simulink subsystem "multi_vehicle_test_subsystem"  (R2025a)
settings: Solver=VariableStepAuto  StartTime=0.0  StopTime=10.0  RelTol=1e-3
libraries: dspstat3 x1
settings Model: Creator=sanborkl  LastModifiedBy=admin

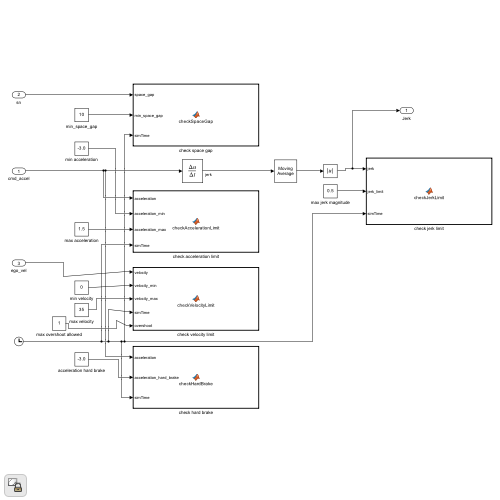
[thumbnail: Simulink's stored preview of the top-level diagram]
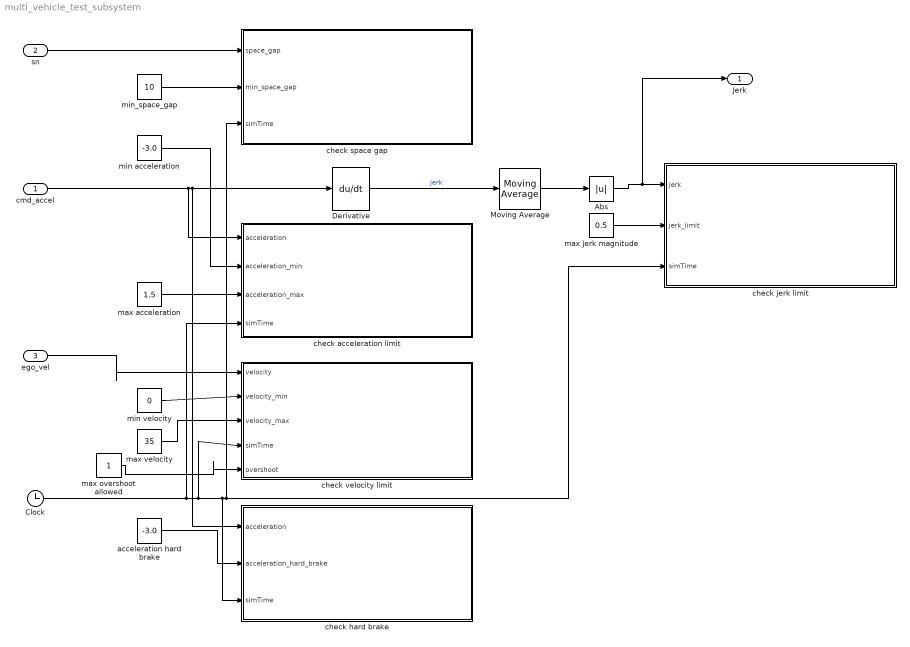
== system multi_vehicle_test_subsystem ==
  cmd_accel : Inport
  sn : Inport  Port=2
  ego_vel : Inport  Port=3
  Abs : Abs  ZeroCross=off  SaturateOnIntegerOverflow=off
  Clock : Clock
  Derivative : Derivative
  Moving Average : dspstat3/Moving Average  Method=Sliding window  ForgettingFactorPort=off  SpecifyWindowLength=on  WindowLength=10  OverlapLength=9  AllowArbitraryInputLength=off  ForgettingFactor=0.9  SimulateUsing=Interpreted execution
  acceleration hard brake : Constant  Value=-3.0
  check acceleration limit : MATLAB Function  TreatAsAtomicUnit=on
  check hard brake : MATLAB Function  TreatAsAtomicUnit=on
  check jerk limit : MATLAB Function  TreatAsAtomicUnit=on
  check space gap : MATLAB Function  TreatAsAtomicUnit=on
  check velocity limit : MATLAB Function  TreatAsAtomicUnit=on
  max acceleration : Constant  Value=1.5
  max jerk magnitude : Constant  Value=0.5
  max overshoot allowed : Constant
  max velocity : Constant  Value=35
  min acceleration : Constant  Value=-3.0
  min velocity : Constant  Value=0
  min_space_gap : Constant  Value=10
  Jerk : Outport
  wires:
  Moving Average/1 -> Abs/1
  min acceleration/1 -> check acceleration limit/2(acceleration_min)
  min_space_gap/1 -> check space gap/2(min_space_gap)
  Clock/1 -> check space gap/3(simTime), check jerk limit/3(simTime), check hard brake/3(simTime), check velocity limit/4(simTime), check acceleration limit/4(simTime)
  sn/1 -> check space gap/1(space_gap)
  ego_vel/1 -> check velocity limit/1(velocity)
  cmd_accel/1 -> Derivative/1, check hard brake/1(acceleration), check acceleration limit/1(acceleration)
  Derivative/1 -> Moving Average/1  "jerk"
  Abs/1 -> Jerk/1, check jerk limit/1(jerk)
  acceleration hard brake/1 -> check hard brake/2(acceleration_hard_brake)
  max acceleration/1 -> check acceleration limit/3(acceleration_max)
  max velocity/1 -> check velocity limit/3(velocity_max)
  min velocity/1 -> check velocity limit/2(velocity_min)
  max jerk magnitude/1 -> check jerk limit/2(jerk_limit)
  max overshoot allowed/1 -> check velocity limit/5(overshoot)

== matlab function multi_vehicle_test_subsystem/check jerk limit ==
  data: jerk input; jerk_limit input; simTime input
function checkJerkLimit(jerk, jerk_limit, simTime)
%#codegen
coder.extrinsic('disp', 'sprintf');

if abs(jerk) > jerk_limit
    msg = sprintf('Warning: Jerk exceeded limit: %.3f > %.3f at t=%.3f', ...
                  abs(jerk), jerk_limit, simTime);
    disp(msg);
end
end

== matlab function multi_vehicle_test_subsystem/check acceleration limit ==
  data: acceleration input; acceleration_min input; acceleration_max input; simTime input
function checkAccelerationLimit(acceleration, acceleration_min, acceleration_max, simTime)
%#codegen
coder.extrinsic('disp', 'sprintf');

if acceleration < acceleration_min || acceleration > acceleration_max
    msg = sprintf('Warning: Acceleration outside allowed bounds: %.3f at t=%.3f', ...
                  acceleration,  simTime);
    disp(msg);
end
end

== matlab function multi_vehicle_test_subsystem/check hard brake ==
  data: acceleration input; acceleration_hard_brake input; simTime input
function checkHardBrake(acceleration, acceleration_hard_brake, simTime)
%#codegen
coder.extrinsic('disp', 'sprintf');

if acceleration <= acceleration_hard_brake
    msg = sprintf('Warning: Hard brake detected: %.3f at t=%.3f', ...
                  acceleration,  simTime);
    disp(msg);
end
end

== matlab function multi_vehicle_test_subsystem/check space gap ==
  data: space_gap input; min_space_gap input; simTime input
function checkSpaceGap(space_gap, min_space_gap, simTime)
%#codegen
coder.extrinsic('disp', 'sprintf');

if (space_gap < min_space_gap) && (space_gap > 0)
    msg = sprintf('Warning: Space gap too close: %.3f at t=%.3f', ...
                  space_gap,  simTime);
    disp(msg);
elseif space_gap <= 0
    msg = sprintf('Error: Space gap violation: %.3f at t=%.3f', ...
                  space_gap,  simTime);
    disp(msg);
end
end

== matlab function multi_vehicle_test_subsystem/check velocity limit ==
  data: velocity input; velocity_min input; velocity_max input; simTime input; overshoot input
function checkVelocityLimit(velocity, velocity_min, velocity_max, simTime, overshoot)

%#codegen
coder.extrinsic('disp', 'sprintf');

if (velocity_max < velocity) && (velocity <= (velocity_max + overshoot))
    msg = sprintf('Warning: Velocity slightly outside allowed bounds: %.3f at t=%.3f', ...
                  velocity,  simTime);
    disp(msg);

elseif velocity < velocity_min && (velocity >= (velocity_min - overshoot))
    msg = sprintf('Warning: Velocity slightly outside allowed bounds: %.3f at t=%.3f', ...
                  velocity,  simTime);
    disp(msg);
 
elseif velocity < velocity_min || velocity > (velocity_max + overshoot)
    msg = sprintf('Error: Velocity outside allowed bounds: %.3f at t=%.3f', ...
                  velocity,  simTime);
    disp(msg);
end
end
